simulink model "Inverse_solution"  (R2023b)
settings: Solver=ode4  StartTime=0.0  StopTime=7  FixedStep=0.0001  RelTol=1e-3
settings Model: Creator=ZLX  LastModifiedBy=ZLX

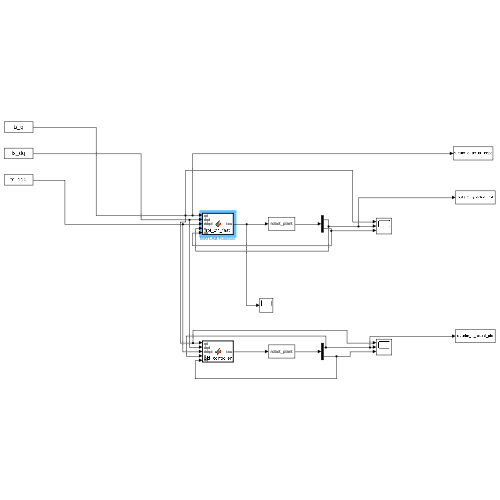
[thumbnail: Simulink's stored preview of the top-level diagram]
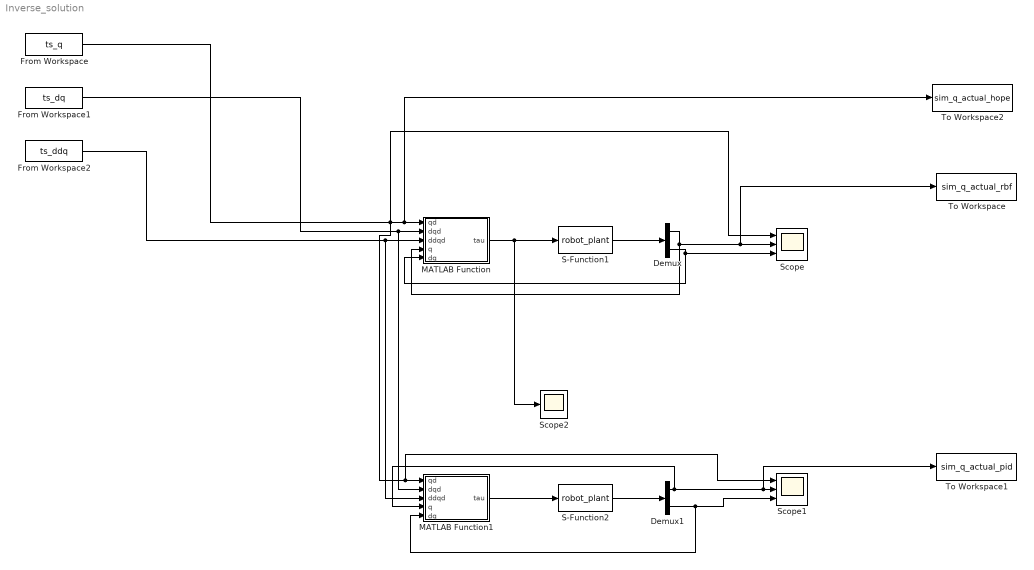
== system Inverse_solution ==
  Demux : Demux  Outputs=[3 3]
  Demux1 : Demux  Outputs=[3 3]
  From Workspace : FromWorkspace  VariableName=ts_q  SampleTime=-1
  From Workspace1 : FromWorkspace  VariableName=ts_dq  SampleTime=-1
  From Workspace2 : FromWorkspace  VariableName=ts_ddq  SampleTime=-1
  MATLAB Function : MATLAB Function  TreatAsAtomicUnit=on
  MATLAB Function1 : MATLAB Function  TreatAsAtomicUnit=on
  S-Function1 : S-Function  FunctionName=robot_plant  SFunctionDeploymentMode=off  EnableBusSupport=off
  S-Function2 : S-Function  FunctionName=robot_plant  SFunctionDeploymentMode=off  EnableBusSupport=off
  Scope : Scope  NumInputPorts=3
  Scope1 : Scope  NumInputPorts=3
  Scope2 : Scope
  To Workspace : ToWorkspace  VariableName=sim_q_actual_rbf  SaveFormat=Timeseries  SampleTime=-1
  To Workspace1 : ToWorkspace  VariableName=sim_q_actual_pid  SaveFormat=Timeseries  SampleTime=-1
  To Workspace2 : ToWorkspace  VariableName=sim_q_actual_hope  SaveFormat=Timeseries  SampleTime=-1
  wires:
  From Workspace2/1 -> MATLAB Function/3(ddqd), MATLAB Function1/3(ddqd)
  Demux/2 -> MATLAB Function/5(dq), Scope/3
  Demux/1 -> MATLAB Function/4(q), To Workspace/1, Scope/2
  MATLAB Function/1(tau) -> S-Function1/1, Scope2/1
  S-Function1/1 -> Demux/1
  From Workspace1/1 -> MATLAB Function1/2(dqd), MATLAB Function/2(dqd)
  From Workspace/1 -> To Workspace2/1, MATLAB Function/1(qd), Scope/1, Scope1/1, MATLAB Function1/1(qd)
  MATLAB Function1/1(tau) -> S-Function2/1
  S-Function2/1 -> Demux1/1
  Demux1/1 -> MATLAB Function1/4(q), To Workspace1/1, Scope1/2
  Demux1/2 -> MATLAB Function1/5(dq), Scope1/3

== matlab function Inverse_solution/MATLAB Function1 ==
  settings: updateMethod=DISCRETE
  data: qd input; tau output; dqd input; ddqd input; q input; dq input
function tau = pid_controller(qd, dqd, ddqd, q, dq)
% PID Controller for Comparison
% 输入接口保持与 RBF 控制器一致，方便直接替换

% --- 1. 定义状态变量 ---
persistent error_sum
if isempty(error_sum)
    error_sum = zeros(3,1); % 积分项累加器
end

% --- 2. PID 参数整定 (经验值) ---
% 这里的参数需要调得比较大才能跟上 RBF 的效果
% 针对关节 1 (基座), 2 (肩), 3 (肘) 分别设置
Kp = diag([500, 500, 500]);  % 比例增益：决定“力气”有多大
Ki = diag([200, 200, 200]);  % 积分增益：消除静差 (抵抗重力)
Kd = diag([20, 20, 20]);     % 微分增益：提供阻尼 (防止震荡)

% --- 3. 计算误差 ---
e = qd - q;       % 位置误差
de = dqd - dq;    % 速度误差

% --- 4. 积分计算 (抗饱和) ---
dt = 0.0001; % 必须与 Simulink Solver 步长一致！(如果你是 0.0001 请修改这里)
error_sum = error_sum + e * dt;

% 积分限幅 (Anti-windup)：防止误差累积过大导致超调
limit_I = 20; 
error_sum = max(min(error_sum, limit_I), -limit_I);

% --- 5. 计算输出力矩 ---
% 标准 PID 公式: tau = Kp*e + Ki*sum + Kd*de
tau = Kp*e + Ki*error_sum + Kd*de;

% --- 6. 输出限幅 ---
tau = max(min(tau, 1000), -1000); % 与 RBF 保持一致的物理限制

end

== matlab function Inverse_solution/MATLAB Function ==
  settings: updateMethod=DISCRETE
  data: qd input; tau output; dqd input; ddqd input; q input; dq input
function tau = rbf_ctrl_fast(qd, dqd, ddqd, q, dq)
% MATLAB Function: 高性能 RBF-SMC 控制器
% 配置: Lambda=80, Gamma=500, Kv=120, dt=0.1ms
% --- 1. 参数定义 ---
persistent W_hat 
persistent Centers
% 初始化
if isempty(W_hat)
    W_hat = zeros(30, 1); 
    Centers = zeros(6, 10);
    for j = 1:10
        Centers(:,j) = (j - 10/2) * 0.5; 
    end
end

% --- 2. 误差计算 ---
e = qd - q;
de = dqd - dq;
Lambda = diag([80, 80, 80]); 
s = de + Lambda * e;

% --- 3. RBF 激活 ---
Z = [e; de]; 
B_width = 0.8;
h = zeros(10, 1);
for j = 1:10
    dist = norm(Z - Centers(:,j))^2;
    h(j) = exp(-dist / (2 * B_width^2));
end

% --- 4. 权重自适应 ---
Gamma = 500; 
W_matrix = reshape(W_hat, 10, 3);

if norm(s) < 0.0001
    dW_matrix = zeros(10, 3);
else
    dW_matrix = Gamma * (h * s');
end

% 离散积分
% ⚠️ 务必确保 Simulink Solver Fixed-step size = 0.0001
dt = 0.0001; 
W_matrix = W_matrix + dW_matrix * dt;
W_hat = W_matrix(:);

% --- 5. 控制输出 ---
f_hat = W_matrix' * h; 


Kv = diag([120, 120, 120]); 
M_approx = diag([2.0, 1.5, 1.0]); 

dqr = dqd + Lambda * e;
ddqr = ddqd + Lambda * de;

tau = M_approx * ddqr + Kv * s + f_hat; 

% 限幅 (防止高增益导致瞬间输出饱和过久)
tau = max(min(tau, 1000), -1000); % 稍微放宽限幅以允许高刚度瞬间出力

end
